simulink model "LQR_Control"  (R2021a)
settings: Solver=VariableStepAuto  StartTime=0.0  StopTime=100  RelTol=1e-3
undefined symbols (not defined in the file): A_m, B_m, C_m, D_m, Earth, K_1, K_2, K_3, WGS84
libraries: aerolibtransform2 x1, aerolibfltsims x1
settings Model: Creator=d3fault  LastModifiedBy=d3fault

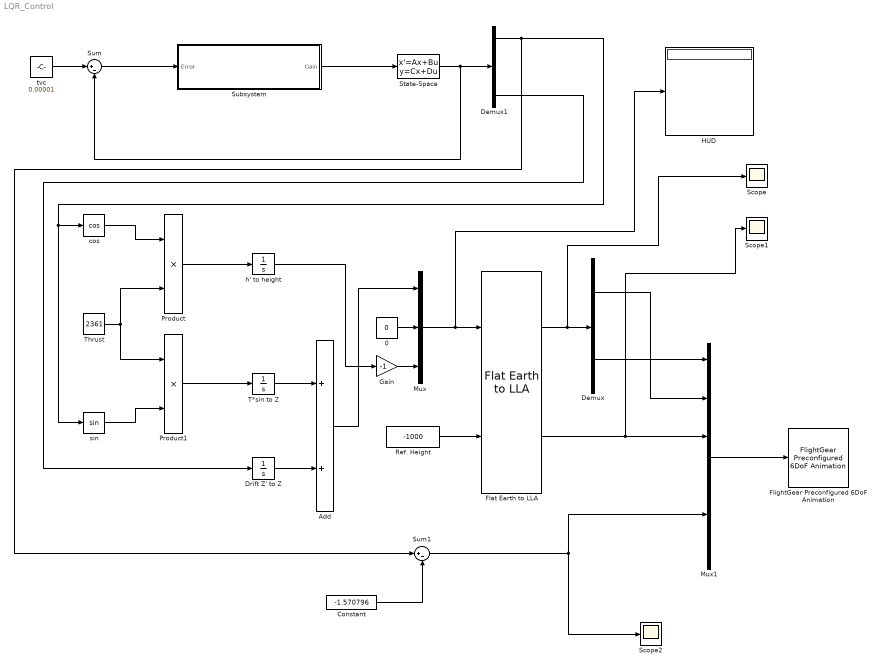
== system LQR_Control ==
  0 : Constant  Value=0
  Add : Sum
  Constant : Constant  Value=-1.570796
  Demux : Demux  Outputs=2
  Demux1 : Demux  Outputs=3
  Drift Z' to Z : Integrator
  Flat Earth to LLA : aerolibtransform2/Flat Earth to LLA  units=Metric (MKS)  ptype=Earth (WGS84)  F=1/298.257223563  R=6378137  refPosPort=off  LL0=[0 10]  psi=0
  FlightGear Preconfigured 6DoF Animation : aerolibfltsims/FlightGear Preconfigured 6DoF Animation  xFlightGearVersion=v2019.1  DestinationIpAddress=127.0.0.1  DestinationPort=5502  SampleTime=1/30  packetVersion=24
  Gain : Gain  Gain=-1
  HUD : Display
  Mux : Mux  Inputs=3
  Mux1 : Mux  Inputs=6
  Product : Product
  Product1 : Product
  Ref. Height : Constant  Value=-1000
  Scope : Scope
  Scope1 : Scope
  Scope2 : Scope
  State-Space : StateSpace  A=A_m  B=B_m  C=C_m  D=D_m  InitialCondition=[0.2; 0; 0]
  Subsystem : Subsystem
  Sum : Sum  Inputs=|+-
  Sum1 : Sum  Inputs=|+-
  T*sin to Z : Integrator
  Thrust : Constant  Value=2361
  "cos " : Trigonometry  Operator=cos
  h' to height : Integrator
  sin : Trigonometry
  tvc : Constant  Value=0.00001
  wires:
  tvc/1 -> Sum/1
  State-Space/1 -> Sum/2, Demux1/1
  Sum/1 -> Subsystem/1(Error)
  Subsystem/1(Gain) -> State-Space/1
  "cos "/1 -> Product/1
  sin/1 -> Product1/2
  Thrust/1 -> Product/2, Product1/1
  Product/1 -> h' to height/1
  Product1/1 -> T*sin to Z/1
  Demux1/3 -> Drift Z' to Z/1
  Drift Z' to Z/1 -> Add/2
  T*sin to Z/1 -> Add/1
  h' to height/1 -> Gain/1
  Gain/1 -> Mux/3
  0/1 -> Mux/2
  Add/1 -> Mux/1
  Ref. Height/1 -> Flat Earth to LLA/2
  Mux/1 -> HUD/1, Flat Earth to LLA/1
  Flat Earth to LLA/1 -> Scope/1, Demux/1
  Demux/1 -> Mux1/2
  Demux/2 -> Mux1/1
  Flat Earth to LLA/2 -> Mux1/3, Scope1/1
  Demux1/1 -> sin/1, "cos "/1, Sum1/1
  Sum1/1 -> Scope2/1, Mux1/5
  Constant/1 -> Sum1/2
  Mux1/1 -> FlightGear Preconfigured 6DoF Animation/1

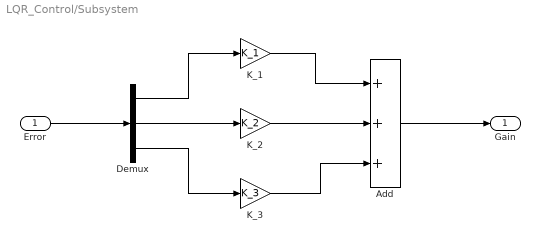
== system LQR_Control/Subsystem ==
  Error : Inport
  Add : Sum  Inputs=+++
  Demux : Demux  Outputs=3
  K_1 : Gain  Gain=K_1
  K_2 : Gain  Gain=K_2
  K_3 : Gain  Gain=K_3
  Gain : Outport
  wires:
  Demux/2 -> K_2/1
  Demux/1 -> K_1/1
  Error/1 -> Demux/1
  Demux/3 -> K_3/1
  K_2/1 -> Add/2
  K_3/1 -> Add/3
  K_1/1 -> Add/1
  Add/1 -> Gain/1
